simulink model "sat_angular_vel"  (R2013b)
settings: Solver=ode45  StartTime=0.0  StopTime=10  RelTol=1e-3
values from neighbouring files (symbols this model uses):
  b = I_free*K_t/nl_speed    (= 1.83906430469e-06)    [parameter_motor.m]
  J_eq = Jw    (= 8.9522375e-05)    [parameter_motor.m]
  Js = 5*Jw    (= 0.000447611875)    [parameter_motor.m]
  Jw = wt_w1*10^-3/2*((dw1/2)^2+(dw2/2)^2)*10^-4    (= 8.9522375e-05)    [parameter_motor.m]
  K_b = (Vm-I_free*R)/nl_speed    (= 0.00979236958951)    [parameter_motor.m]
  K_t = T_stall/I_stall    (= 0.0070615)    [parameter_motor.m]
  L = 0.5    [parameter_motor.m]
  R = 0.001    [kalman_filter.m]    (also in parameter_motor.m = 2.4)
undefined symbols (not defined in the file or in its folder): sigbuilder_block
libraries: simulink x2
settings Model: Creator=sanjay  LastModifiedBy=sanjay

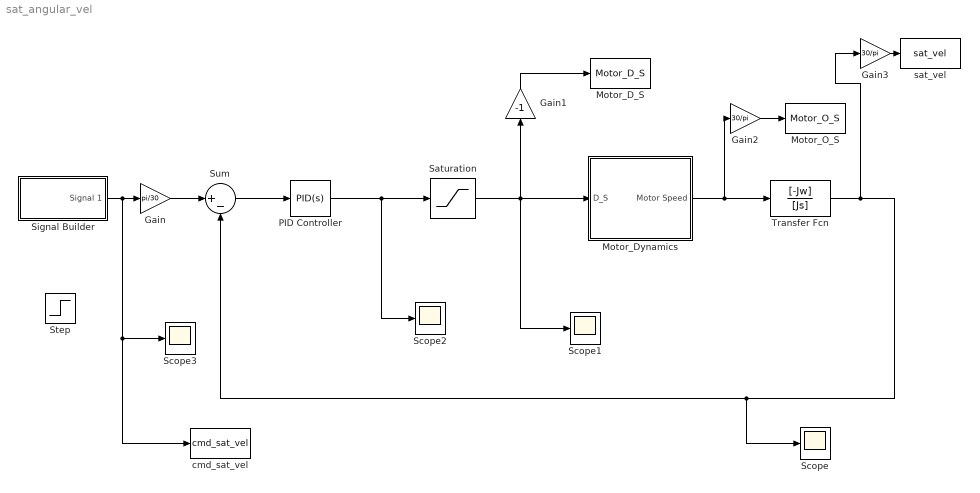
== system sat_angular_vel ==
  Gain : Gain  Gain=pi/30
  Gain1 : Gain  Gain=-1
  Gain2 : Gain  Gain=30/pi
  Gain3 : Gain  Gain=30/pi
  Motor_D_S : ToWorkspace  VariableName=Motor_D_S  SampleTime=-1  SaveFormat=Timeseries
  Motor_Dynamics : Subsystem
  Motor_O_S : ToWorkspace  VariableName=Motor_O_S  SampleTime=-1  SaveFormat=Timeseries
  PID Controller : simulink/Continuous/PID Controller  Controller=PID  TimeDomain=Continuous-time  SampleTime=1  IntegratorMethod=Forward Euler  FilterMethod=Forward Euler  Form=Parallel  P=90.5291625083045  I=871.388896065982  D=1.47943830348446  N=54.5908897983753  InitialConditionSource=internal  InitialConditionForIntegrator=0  InitialConditionForFilter=0  ExternalReset=none  LimitOutput=off  UpperSaturationLimit=inf  LowerSaturationLimit=-inf  LinearizeAsGain=on  AntiWindupMode=none  Kb=1  TrackingMode=off  Kt=1  PParamMin=[]  PParamMax=[]  IParamMin=[]  IParamMax=[]  DParamMin=[]  DParamMax=[]  NParamMin=[]  NParamMax=[]  KbParamMin=[]  KbParamMax=[]  KtParamMin=[]  KtParamMax=[]  POutMin=[]  POutMax=[]  IOutMin=[]  IOutMax=[]  DOutMin=[]  DOutMax=[]  NOutMin=[]  NOutMax=[]  KbOutMin=[]  KbOutMax=[]  KtOutMin=[]  KtOutMax=[]  IntegratorOutMin=[]  IntegratorOutMax=[]  FilterOutMin=[]  FilterOutMax=[]  SumOutMin=[]  SumOutMax=[]  SumI1OutMin=[]  SumI1OutMax=[]  SumI2OutMin=[]  SumI2OutMax=[]  SumI3OutMin=[]  SumI3OutMax=[]  SumDOutMin=[]  SumDOutMax=[]  SaturationOutMin=[]  SaturationOutMax=[]  IntegratorContinuousStateAttributes=''  IntegratorStateMustResolveToSignalObject=off  IntegratorRTWStateStorageClass=Auto  FilterContinuousStateAttributes=''  FilterStateMustResolveToSignalObject=off  FilterRTWStateStorageClass=Auto
  Saturation : Saturate  UpperLimit=7800  LowerLimit=-7800
  Scope{,1..3} (4 alike) : Scope
      Scope2 settings: SaveName=ScopeData2
      Scope3 settings: SaveName=ScopeData3
  Signal Builder : Subsystem  Tag=STV Subsys  LoadFcn=sigbuilder_block('load');  StartFcn=sigbuilder_block('start');  StopFcn=sigbuilder_block('stop');  ClipboardFcn=sigbuilder_block('clipboard');  mask(Sigbuilder block){}
      mask help: Simulink:masks:SigbuilderBlock_MD
      mask init:
      | if ~strcmp(get_param(bdroot(gcbh),'SimulationStatus'),'stopped') tuvar = sigbuilder_block('maskInit'); end
      settings: CopyFcn=sigbuilder_block('copy');  DeleteFcn=sigbuilder_block('delete');  ModelCloseFcn=sigbuilder_block('modelClose');  PreSaveFcn=sigbuilder_block('preSave');  PauseFcn=sigbuilder_block('pause');  ContinueFcn=sigbuilder_block('continue');  NameChangeFcn=sigbuilder_block('namechange');  OpenFcn=sigbuilder_block('open',[159 97.5 550.5 394.5 ]);  CloseFcn=sigbuilder_block('close');
      mask Display: plot(0, 0, 100, 100,[2, 2, 32, 32, 2], [68, 8, 8, 68, 68],[32, 2], [38, 38], [32, 19, 2],[53, 60, 44], [32, 17, 17, 2],[16, 16, 31, 31]);txt = getActiveGroup(gcbh);text(2, 100, txt,'verticalAlignment', 'top');
  Step : Step  After=30  SampleTime=0
  Sum : Sum  Inputs=|+-
  Transfer Fcn : TransferFcn  Numerator=[-Jw]  Denominator=[Js]
  cmd_sat_vel : ToWorkspace  VariableName=cmd_sat_vel  SampleTime=-1  SaveFormat=Timeseries
  sat_vel : ToWorkspace  VariableName=sat_vel  SampleTime=-1  SaveFormat=Timeseries
  wires:
  Saturation/1 -> Scope1/1, Gain1/1, Motor_Dynamics/1(D_S)
  Motor_Dynamics/1(Motor Speed) -> Gain2/1, Transfer Fcn/1
  Sum/1 -> PID Controller/1
  Transfer Fcn/1 -> Gain3/1, Scope/1, Sum/2
  Gain/1 -> Sum/1
  PID Controller/1 -> Scope2/1, Saturation/1
  Signal Builder/1(Signal 1) -> cmd_sat_vel/1, Scope3/1, Gain/1
  Gain3/1 -> sat_vel/1
  Gain2/1 -> Motor_O_S/1
  Gain1/1 -> Motor_D_S/1

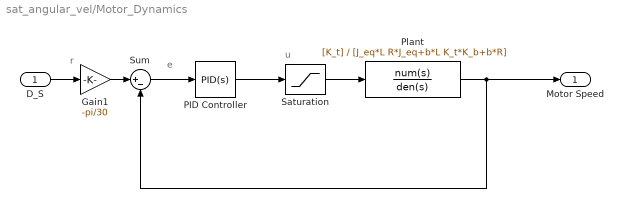
== system sat_angular_vel/Motor_Dynamics ==
  note: u
  note: e
  note: r
  D_S : Inport
  Gain1 : Gain  Gain=-pi/30
  PID Controller : simulink/Continuous/PID Controller  RequirementInfo={'other' '..\controller values.xlsx' '@Simulink_requirement_item_1' 'true' 'iter1' '' ; 'other' '..\controller values.xlsx' '@Simulink_requirement_item_1' 'true' '' '' ; 'other' '..\controller values.xlsx' '@Simulink_requirement_item_2' 'true' '' '' } %GIDa_fbdd2cd8_7785_42e6_8e75_0620455e6e7c  Controller=PID  TimeDomain=Continuous-time  SampleTime=1  IntegratorMethod=Forward Euler  FilterMethod=Forward Euler  Form=Parallel  P=0.428884127030052  I=0.071698956393298  D=0.0413910090495183  N=30.5058365758755  InitialConditionSource=internal  InitialConditionForIntegrator=0  InitialConditionForFilter=0  ExternalReset=none  LimitOutput=off  UpperSaturationLimit=inf  LowerSaturationLimit=-inf  LinearizeAsGain=on  AntiWindupMode=none  Kb=1  TrackingMode=off  Kt=1  PParamMin=[]  PParamMax=[]  IParamMin=[]  IParamMax=[]  DParamMin=[]  DParamMax=[]  NParamMin=[]  NParamMax=[]  KbParamMin=[]  KbParamMax=[]  KtParamMin=[]  KtParamMax=[]  POutMin=[]  POutMax=[]  IOutMin=[]  IOutMax=[]  DOutMin=[]  DOutMax=[]  NOutMin=[]  NOutMax=[]  KbOutMin=[]  KbOutMax=[]  KtOutMin=[]  KtOutMax=[]  IntegratorOutMin=[]  IntegratorOutMax=[]  FilterOutMin=[]  FilterOutMax=[]  SumOutMin=[]  SumOutMax=[]  SumI1OutMin=[]  SumI1OutMax=[]  SumI2OutMin=[]  SumI2OutMax=[]  SumI3OutMin=[]  SumI3OutMax=[]  SumDOutMin=[]  SumDOutMax=[]  SaturationOutMin=[]  SaturationOutMax=[]  IntegratorContinuousStateAttributes=''  IntegratorStateMustResolveToSignalObject=off  IntegratorRTWStateStorageClass=Auto  FilterContinuousStateAttributes=''  FilterStateMustResolveToSignalObject=off  FilterRTWStateStorageClass=Auto
  Plant : TransferFcn  Numerator=[K_t]  Denominator=[J_eq*L R*J_eq+b*L K_t*K_b+b*R]
  Saturation : Saturate  UpperLimit=9  LowerLimit=-9
  Sum : Sum  Inputs=|+-
  Motor Speed : Outport
  wires:
  D_S/1 -> Gain1/1
  Saturation/1 -> Plant/1
  Plant/1 -> Motor Speed/1, Sum/2
  PID Controller/1 -> Saturation/1
  Sum/1 -> PID Controller/1
  Gain1/1 -> Sum/1

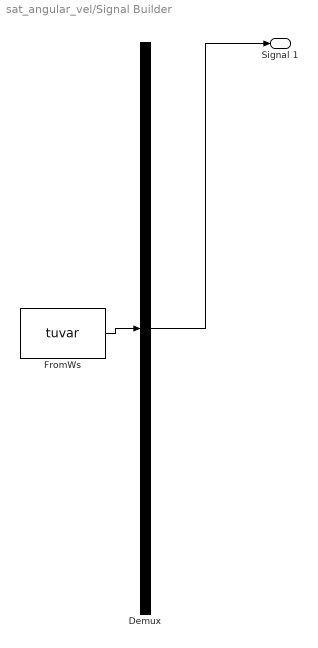
== system sat_angular_vel/Signal Builder ==
  Demux : Demux  Tag=STV Demux  Outputs=1
  FromWs : FromWorkspace  Tag=STV FromWs  VariableName=tuvar  SampleTime=0
      SigBuilderData=|
      | common.afterFinalStr = 'Extrapolate'
      | common.sampleTime = 0
      | dataSet.timeRange = [0 10]
      | dataSet.name = 'Group 1'
      | sbobj.Groups.Name = 'Group 1'
      | sbobj.Groups.Signals.Name = 'Signal 1'
      | sbobj.Groups.Signals.XData = [0 1.02 2 5 10]
      | sbobj.Groups.Signals.YData = [0 30 30 -32.4 0]
  Signal 1 : Outport  Tag=STV Outport
  wires:
  Demux/1 -> Signal 1/1
  FromWs/1 -> Demux/1
